simulink model "SimulationModel"  (R2019b)
settings: Solver=FixedStepAuto  StartTime=0.0  StopTime=simStopTime  FixedStep=Ts  RelTol=1e-3
PostLoadFcn:
  | init
values from neighbouring files (symbols this model uses):
  total_vehicles = evalin('base','total_vehicles')    [VehicleLogicSimulator.m]
  x0 = evalin('base','x0')    [VehicleLogicSimulator.m]
  y0 = evalin('base','y0')    [VehicleLogicSimulator.m]
  yaw0 = evalin('base','yaw0')    [VehicleLogicSimulator.m]
undefined symbols (not defined in the file or in its folder): Cf, Cr, index_show_car, Iz, lf, longitudinal_velocity, lr, m, position, tau, Ts, v0, velocity, yaw_angle, yaw_rate
libraries: autolibshared x3, drivingscenarioandsensors x1, simulink_extras x1
settings Model: Creator=The MathWorks, Inc.  LastModifiedBy=curtm
settings DataIOCC: ReturnWorkspaceOutputs=off
settings DebuggingCC: ParameterPrecisionLossMsg=none  PregeneratedLibrarySubsystemCodeDiagnostic=none  ArithmeticOperatorsInVariantConditions=warning
settings HardwareCC: ProdLongLongMode=on
settings SFSimCC: SimUseLocalCustomCode=off  CustomCodeUndefinedFunction=UseInterfaceOnly
settings RTWCC: RTWUseLocalCustomCode=off

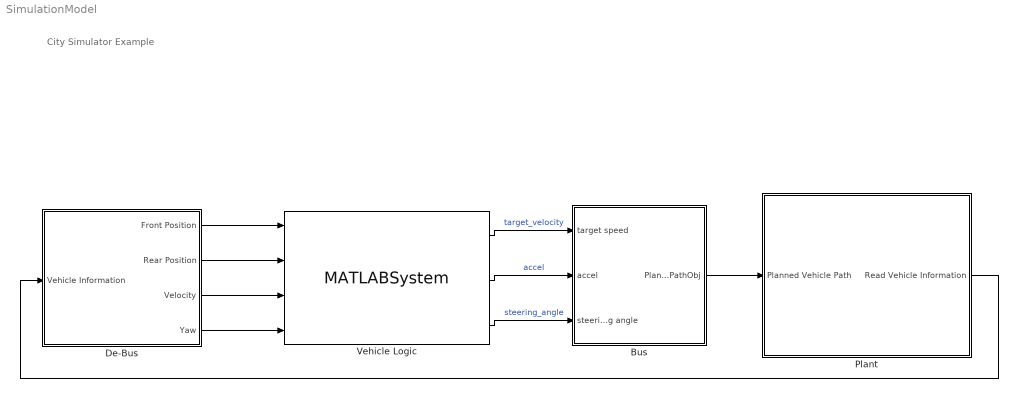
== system SimulationModel ==
  note: City Simulator Example
  Bus : Subsystem
  De-Bus : Subsystem
  Plant : Subsystem
  Vehicle Logic : MATLABSystem  System=VehicleLogicMatlabSystem  SimulateUsing=Code generation
      mask Type: VehicleLogicMatlabSystem
      mask Display:
      | disp('VehicleLogicMatlabSystem');
      | port_label('input',1,'front_pos');
      | port_label('input',2,'rear_pos');
      | port_label('input',3,'velocities');
      | port_label('input',4,'yaws');
      | port_label('output',1,'target_speed');
      | port_label('output',2,'accel');
      | port_label('output',3,'streering_angle');
  wires:
  Bus/1(PlannedVehiclePathObj) -> Plant/1(Planned Vehicle Path)
  Vehicle Logic/1 -> Bus/1(target speed)  "target_velocity"
  Vehicle Logic/2 -> Bus/2(accel)  "accel"
  Vehicle Logic/3 -> Bus/3(steering angle)  "steering_angle"
  De-Bus/2(Rear Position) -> Vehicle Logic/2
  De-Bus/3(Velocity) -> Vehicle Logic/3
  De-Bus/4(Yaw) -> Vehicle Logic/4
  Plant/1(Read Vehicle Information) -> De-Bus/1(Vehicle Information)
  De-Bus/1(Front Position) -> Vehicle Logic/1

== system SimulationModel/Bus ==
  target speed : Inport  OutDataTypeStr=double
  accel : Inport  Port=2  OutDataTypeStr=double
  steering angle : Inport  Port=3  OutDataTypeStr=double
  Planned Vehicle Path From Index 1 : Subsystem  mask{index=1, size=total_vehicles}
      mask prompts: index "Which element of the array?"; size "How many AVs are there?"
  Planned Vehicle Path From Index 2 : Subsystem  mask{index=2, size=total_vehicles}
      mask prompts: index "Which element of the array?"; size "How many AVs are there?"
  Vector Concatenate : Concatenate
  PlannedVehiclePathObj : Outport  OutDataTypeStr=Bus: PlannedVehicleDynamics
  wires:
  Vector Concatenate/1 -> PlannedVehiclePathObj/1
  Planned Vehicle Path From Index 1/1(PlannedVehiclePathObj) -> Vector Concatenate/1
  target speed/1 -> Planned Vehicle Path From Index 2/1(target_speed), Planned Vehicle Path From Index 1/1(target_speed)
  accel/1 -> Planned Vehicle Path From Index 2/2(accel), Planned Vehicle Path From Index 1/2(accel)
  steering angle/1 -> Planned Vehicle Path From Index 2/3(steering_angle), Planned Vehicle Path From Index 1/3(steering_angle)
  Planned Vehicle Path From Index 2/1(PlannedVehiclePathObj) -> Vector Concatenate/2

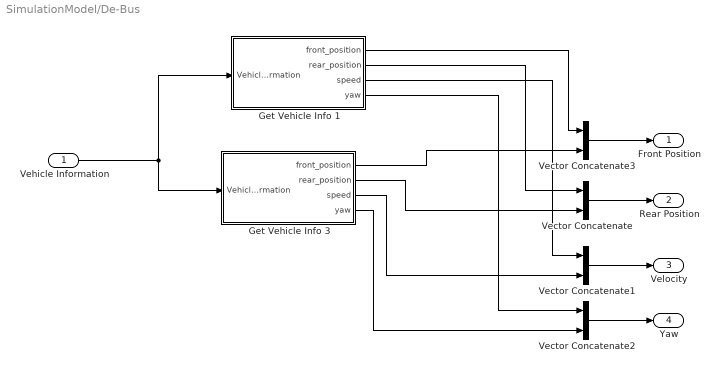
== system SimulationModel/De-Bus ==
  Vehicle Information : Inport
  Get Vehicle Info 1 : Subsystem  mask{index=1, size=total_vehicles}
  Get Vehicle Info 3 : Subsystem  mask{index=2, size=total_vehicles}
  Vector Concatenate{,1..3} (4 alike) : Concatenate
  Front Position : Outport
  Rear Position : Outport  Port=2
  Velocity : Outport  Port=3
  Yaw : Outport  Port=4
  wires:
  Vector Concatenate/1 -> Rear Position/1
  Vector Concatenate1/1 -> Velocity/1
  Vehicle Information/1 -> Get Vehicle Info 3/1(Vehicle Information), Get Vehicle Info 1/1(Vehicle Information)
  Get Vehicle Info 1/2(rear_position) -> Vector Concatenate/1
  Get Vehicle Info 1/3(speed) -> Vector Concatenate1/1
  Get Vehicle Info 3/2(rear_position) -> Vector Concatenate/2
  Get Vehicle Info 3/3(speed) -> Vector Concatenate1/2
  Vector Concatenate2/1 -> Yaw/1
  Get Vehicle Info 1/4(yaw) -> Vector Concatenate2/1
  Get Vehicle Info 3/4(yaw) -> Vector Concatenate2/2
  Get Vehicle Info 1/1(front_position) -> Vector Concatenate3/1
  Vector Concatenate3/1 -> Front Position/1
  Get Vehicle Info 3/1(front_position) -> Vector Concatenate3/2

== system SimulationModel/Plant ==
  note: Vehicle and Environment
  Planned Vehicle Path : Inport  OutDataTypeStr=Bus: PlannedVehicleDynamics  SampleTime=Ts
  Pack for Scenario Reader : Subsystem
  Scenario Reader : drivingscenarioandsensors/Scenario Reader  ScenarioSource=From file  ScenarioFileName=MarcCity.mat  ScenarioVariableName=scenario  OutputCoordinateSystem=Vehicle coordinates  EgoVehicleSource=Input port  EgoVehicleActorID=1  SampleTime=Ts  LaneBoundaryOutput=Ego vehicle lane boundaries  LaneBoundaryDistance=0:0.5:60  LaneBoundaryLocation=Inner edge of lane markings  BusNameSource=Auto  BusName=BusActors  BusName2Source=Auto  BusName2=BusLaneBoundaries  SimulateUsing=Interpreted execution
      settings: SourceProductName=Automated Driving Toolbox
  Terminator : Terminator
  Terminator1 : Terminator
  Vehicle Simulation : Subsystem
  Vehicle Simulation1 : Subsystem  Commented=on  TreatAsAtomicUnit=on
  Read Vehicle Information : Outport  SampleTime=Ts
  wires:
  Planned Vehicle Path/1 -> Vehicle Simulation/1(Planned Vehicle Dynamics)
  Vehicle Simulation/1(Next Vehicle Dynamics) -> Pack for Scenario Reader/1(Bus), Read Vehicle Information/1
  Scenario Reader/1 -> Terminator/1
  Scenario Reader/2 -> Terminator1/1
  Pack for Scenario Reader/1(Scenario Reader Struct) -> Scenario Reader/1

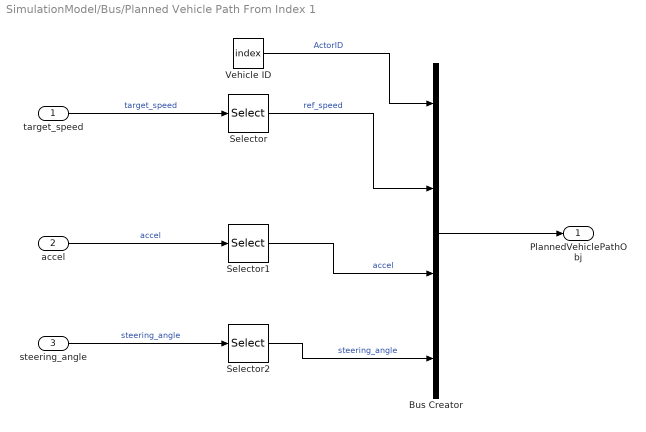
== system SimulationModel/Bus/Planned Vehicle Path From Index 1 ==
  target_speed : Inport
  accel : Inport  Port=2
  steering_angle : Inport  Port=3
  Bus Creator : BusCreator  Inputs=4  OutDataTypeStr=Bus: PlannedVehicleDynamics  NonVirtualBus=on
  Selector : Selector  NumberOfDimensions=2  InputPortWidth=size  IndexOptions=Index vector (dialog),Index vector (dialog)  Indices=index,1  OutputSizes=1,1
  Selector1 : Selector  NumberOfDimensions=2  InputPortWidth=size  IndexOptions=Index vector (dialog),Index vector (dialog)  Indices=index,1  OutputSizes=1,1
  Selector2 : Selector  NumberOfDimensions=2  InputPortWidth=size  IndexOptions=Index vector (dialog),Index vector (dialog)  Indices=index,1  OutputSizes=1,1
  Vehicle ID : Constant  Value=index
  PlannedVehiclePathObj : Outport
  wires:
  target_speed/1 -> Selector/1  "target_speed"
  steering_angle/1 -> Selector2/1  "steering_angle"
  accel/1 -> Selector1/1  "accel"
  Selector/1 -> Bus Creator/2  "ref_speed"
  Selector1/1 -> Bus Creator/3  "accel"
  Selector2/1 -> Bus Creator/4  "steering_angle"
  Bus Creator/1 -> PlannedVehiclePathObj/1
  Vehicle ID/1 -> Bus Creator/1  "ActorID"

== system SimulationModel/Bus/Planned Vehicle Path From Index 2 ==
  target_speed : Inport
  accel : Inport  Port=2
  steering_angle : Inport  Port=3
  Bus Creator : BusCreator  Inputs=4  OutDataTypeStr=Bus: PlannedVehicleDynamics  NonVirtualBus=on
  Selector : Selector  InputPortWidth=size  IndexOptions=Index vector (dialog)  Indices=index  OutputSizes=1
  Selector3 : Selector  InputPortWidth=size  IndexOptions=Index vector (dialog)  Indices=index  OutputSizes=1
  Selector4 : Selector  InputPortWidth=size  IndexOptions=Index vector (dialog)  Indices=index  OutputSizes=1
  Vehicle ID : Constant  Value=index
  PlannedVehiclePathObj : Outport
  wires:
  target_speed/1 -> Selector/1  "target_speed"
  steering_angle/1 -> Selector4/1  "steering_angle"
  accel/1 -> Selector3/1  "accel"
  Selector/1 -> Bus Creator/2  "ref_speed"
  Selector3/1 -> Bus Creator/3  "accel"
  Selector4/1 -> Bus Creator/4  "steering_angle"
  Bus Creator/1 -> PlannedVehiclePathObj/1
  Vehicle ID/1 -> Bus Creator/1  "ActorID"

== system SimulationModel/De-Bus/Get Vehicle Info 1 ==
  Vehicle Information : Inport  OutDataTypeStr=Bus: NextVehicleDynamics
  Bus Selector : BusSelector  OutputSignals=front_position,rear_position,longitudinal_velocity,yaw_angle
  Selector : Selector  InputPortWidth=size  IndexOptions=Index vector (dialog)  Indices=[index]  OutputSizes=1
  front_position : Outport
  rear_position : Outport  Port=2
  speed : Outport  Port=3
  yaw : Outport  Port=4
  wires:
  Vehicle Information/1 -> Selector/1
  Selector/1 -> Bus Selector/1
  Bus Selector/2 -> rear_position/1  "<rear_position>"
  Bus Selector/3 -> speed/1  "<longitudinal_velocity>"
  Bus Selector/4 -> yaw/1  "<yaw_angle>"
  Bus Selector/1 -> front_position/1  "<front_position>"

== system SimulationModel/De-Bus/Get Vehicle Info 3 ==
  Vehicle Information : Inport  OutDataTypeStr=Bus: NextVehicleDynamics
  Bus Selector : BusSelector  OutputSignals=front_position,rear_position,longitudinal_velocity,yaw_angle
  Selector : Selector  InputPortWidth=size  IndexOptions=Index vector (dialog)  Indices=[index]  OutputSizes=1
  front_position : Outport
  rear_position : Outport  Port=2
  speed : Outport  Port=3
  yaw : Outport  Port=4
  wires:
  Vehicle Information/1 -> Selector/1
  Selector/1 -> Bus Selector/1
  Bus Selector/2 -> rear_position/1  "<rear_position>"
  Bus Selector/3 -> speed/1  "<longitudinal_velocity>"
  Bus Selector/4 -> yaw/1  "<yaw_angle>"
  Bus Selector/1 -> front_position/1  "<front_position>"

== system SimulationModel/Plant/Pack for Scenario Reader ==
  Bus : Inport
  Clock : Clock  Commented=on
  MATLAB Function : MATLAB Function  Commented=on  TreatAsAtomicUnit=on
  Multiport Switch : MultiPortSwitch  Inputs=2
  Pack bus : Subsystem  mask{index=1, size=total_vehicles}
  Pack bus1 : Subsystem  mask{index=2, size=total_vehicles}
  Selector : Constant  Value=index_show_car
  Terminator : Terminator  Commented=on
  Scenario Reader Struct : Outport
  wires:
  Bus/1 -> Pack bus1/1(Bus), Pack bus/1(Bus)
  Pack bus/1(Scenario Reader Struct) -> Multiport Switch/2
  Multiport Switch/1 -> Scenario Reader Struct/1
  Pack bus1/1(Scenario Reader Struct) -> Multiport Switch/3
  Selector/1 -> Multiport Switch/1
  Clock/1 -> MATLAB Function/3(simTime)
  MATLAB Function/1(Actors) -> Terminator/1

== system SimulationModel/Plant/Vehicle Simulation ==
  Planned Vehicle Dynamics : Inport
  Vector Concatenate : Concatenate
  Vehicle 1 Simulation : Subsystem  mask{index=1, size=total_vehicles}
  Vehicle 2 Simulation : Subsystem  mask{index=2, size=total_vehicles}
  Next Vehicle Dynamics : Outport
  wires:
  Planned Vehicle Dynamics/1 -> Vehicle 2 Simulation/1(InBus), Vehicle 1 Simulation/1(InBus)
  Vehicle 1 Simulation/1(outBus) -> Vector Concatenate/1
  Vector Concatenate/1 -> Next Vehicle Dynamics/1
  Vehicle 2 Simulation/1(outBus) -> Vector Concatenate/2

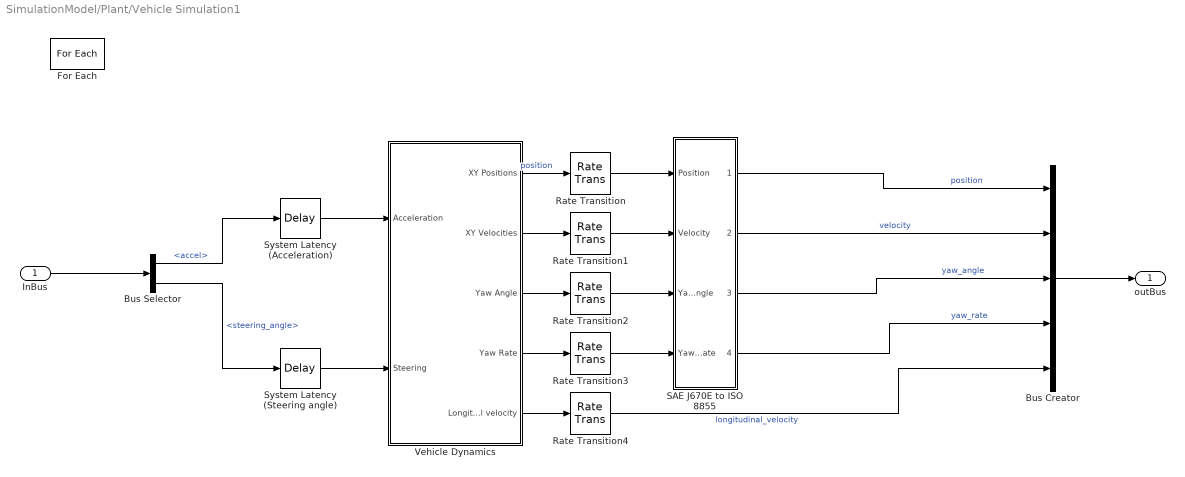
== system SimulationModel/Plant/Vehicle Simulation1 ==
  InBus : Inport  OutDataTypeStr=Bus: PlannedVehicleDynamics  PortDimensions=1  SampleTime=Ts  Partition=on  PartitionDimension=1  PartitionWidth=1  PartitionOffset=0
  Bus Creator : BusCreator  Inputs=position,velocity,yaw_angle,yaw_rate,longitudinal_velocity  OutDataTypeStr=Bus: NextVehicleDynamics  NonVirtualBus=on
  Bus Selector : BusSelector  OutputSignals=accel,steering_angle
  For Each : ForEach  DisableCoverage=on
  Rate Transition{,1..4} (5 alike) : RateTransition  OutPortSampleTime=Ts
  SAE J670E to ISO 8855 : Subsystem
  System Latency (Acceleration) : TransportDelay  DelayTime=Ts
  System Latency (Steering angle) : TransportDelay  DelayTime=Ts
  Vehicle Dynamics : Subsystem  VariantControl=Variant2
  outBus : Outport  OutDataTypeStr=Bus: NextVehicleDynamics  SampleTime=Ts  ConcatenationDimension=1
  wires:
  System Latency (Steering angle)/1 -> Vehicle Dynamics/2(Steering)
  System Latency (Acceleration)/1 -> Vehicle Dynamics/1(Acceleration)
  Vehicle Dynamics/1(XY Positions) -> Rate Transition/1  "position"
  Rate Transition/1 -> SAE J670E to ISO 8855/1(Position)
  Vehicle Dynamics/5(Longitudinal velocity) -> Rate Transition4/1
  SAE J670E to ISO 8855/2(2) -> Bus Creator/2  "velocity"
  Vehicle Dynamics/3(Yaw Angle) -> Rate Transition2/1
  SAE J670E to ISO 8855/1(1) -> Bus Creator/1  "position"
  Rate Transition4/1 -> Bus Creator/5  "longitudinal_velocity"
  SAE J670E to ISO 8855/4(4) -> Bus Creator/4  "yaw_rate"
  Rate Transition3/1 -> SAE J670E to ISO 8855/4(Yaw Rate)
  Rate Transition1/1 -> SAE J670E to ISO 8855/2(Velocity)
  SAE J670E to ISO 8855/3(3) -> Bus Creator/3  "yaw_angle"
  Vehicle Dynamics/2(XY Velocities) -> Rate Transition1/1
  Vehicle Dynamics/4(Yaw Rate) -> Rate Transition3/1
  Rate Transition2/1 -> SAE J670E to ISO 8855/3(Yaw Angle)
  InBus/1 -> Bus Selector/1
  Bus Selector/1 -> System Latency (Acceleration)/1  "<accel>"
  Bus Selector/2 -> System Latency (Steering angle)/1  "<steering_angle>"
  Bus Creator/1 -> outBus/1

== system SimulationModel/Plant/Pack for Scenario Reader/Pack bus ==
  Bus : Inport
  Bus Selector : BusSelector  OutputSignals=rear_position,velocity,yaw_angle,yaw_rate,longitudinal_velocity
  Constant : Constant  Value=index
  Pack Ego Actor : MATLAB Function  TreatAsAtomicUnit=on  SystemSampleTime=Ts
  Selector : Selector  InputPortWidth=size  IndexOptions=Index vector (dialog)  Indices=index  OutputSizes=1
  Terminator : Terminator
  Scenario Reader Struct : Outport
  wires:
  Constant/1 -> Pack Ego Actor/1(actorID)
  Bus Selector/4 -> Pack Ego Actor/5(yawRate)  "<yaw_rate>"
  Bus Selector/3 -> Pack Ego Actor/4(yaw)  "<yaw_angle>"
  Bus Selector/2 -> Pack Ego Actor/3(vel)  "<velocity>"
  Bus Selector/5 -> Terminator/1  "<longitudinal_velocity>"
  Pack Ego Actor/1(a) -> Scenario Reader Struct/1
  Selector/1 -> Bus Selector/1  "bus"
  Bus/1 -> Selector/1
  Bus Selector/1 -> Pack Ego Actor/2(pos)  "<rear_position>"

== system SimulationModel/Plant/Pack for Scenario Reader/Pack bus1 ==
  Bus : Inport
  Bus Selector : BusSelector  OutputSignals=rear_position,velocity,yaw_angle,yaw_rate,longitudinal_velocity
  Constant : Constant  Value=index
  Pack Ego Actor : MATLAB Function  TreatAsAtomicUnit=on  SystemSampleTime=Ts
  Selector : Selector  InputPortWidth=size  IndexOptions=Index vector (dialog)  Indices=index  OutputSizes=1
  Terminator : Terminator
  Scenario Reader Struct : Outport
  wires:
  Constant/1 -> Pack Ego Actor/1(actorID)
  Bus Selector/4 -> Pack Ego Actor/5(yawRate)  "<yaw_rate>"
  Bus Selector/3 -> Pack Ego Actor/4(yaw)  "<yaw_angle>"
  Bus Selector/2 -> Pack Ego Actor/3(vel)  "<velocity>"
  Bus Selector/5 -> Terminator/1  "<longitudinal_velocity>"
  Pack Ego Actor/1(a) -> Scenario Reader Struct/1
  Bus Selector/1 -> Pack Ego Actor/2(pos)  "<rear_position>"
  Selector/1 -> Bus Selector/1  "bus"
  Bus/1 -> Selector/1

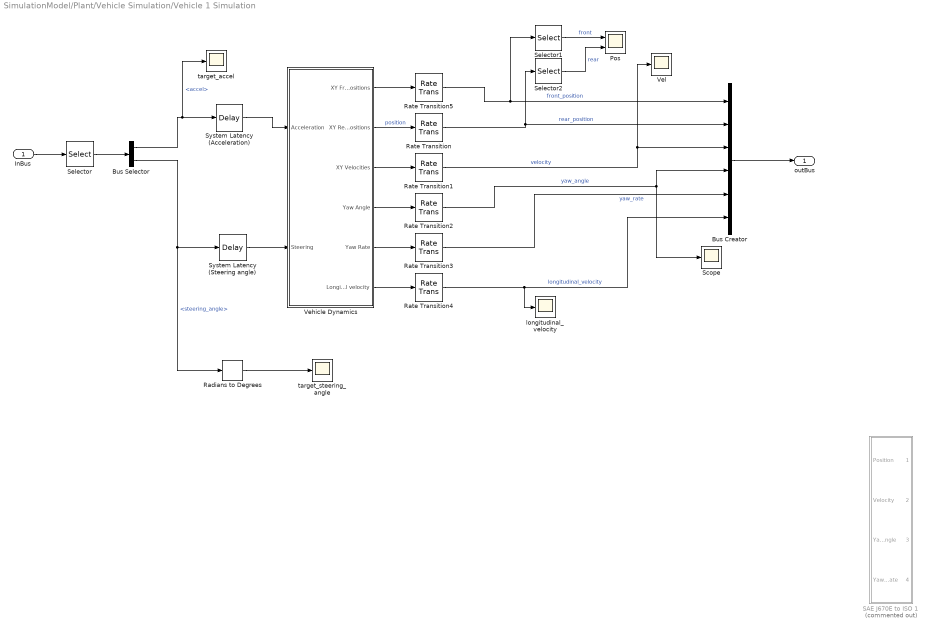
== system SimulationModel/Plant/Vehicle Simulation/Vehicle 1 Simulation ==
  InBus : Inport  OutDataTypeStr=Bus: PlannedVehicleDynamics  PortDimensions=1  SampleTime=Ts
  Bus Creator : BusCreator  Inputs=6  OutDataTypeStr=Bus: NextVehicleDynamics  NonVirtualBus=on
  Bus Selector : BusSelector  OutputSignals=accel,steering_angle
  Pos : Scope  NumInputPorts=2
  Radians to Degrees : simulink_extras/Transformations/Radians to Degrees
  Rate Transition{,1..5} (6 alike) : RateTransition  OutPortSampleTime=Ts
  SAE J670E to ISO 1 : Subsystem  Commented=on
  Scope : Scope
  Selector : Selector  InputPortWidth=size  IndexOptions=Index vector (dialog)  Indices=index  OutputSizes=1
  Selector1 : Selector  InputPortWidth=2  IndexOptions=Index vector (dialog)  Indices=2  OutputSizes=1
  Selector2 : Selector  InputPortWidth=2  IndexOptions=Index vector (dialog)  Indices=2  OutputSizes=1
  System Latency (Acceleration) : TransportDelay  DelayTime=Ts
  System Latency (Steering angle) : TransportDelay  DelayTime=Ts
  Vehicle Dynamics : Subsystem  VariantControl=Variant2
  Vel : Scope
  longitudinal_velocity : Scope
  target_accel : Scope
  target_steering_angle : Scope
  outBus : Outport  OutDataTypeStr=Bus: NextVehicleDynamics  SampleTime=Ts
  wires:
  Rate Transition2/1 -> Scope/1, Bus Creator/4  "yaw_angle"
  Rate Transition4/1 -> Bus Creator/6, longitudinal_velocity/1  "longitudinal_velocity"
  Vehicle Dynamics/6(Longitudinal velocity) -> Rate Transition4/1
  Vehicle Dynamics/4(Yaw Angle) -> Rate Transition2/1
  Vehicle Dynamics/3(XY Velocities) -> Rate Transition1/1
  Vehicle Dynamics/2(XY Rear Positions) -> Rate Transition/1  "position"
  Bus Creator/1 -> outBus/1
  Bus Selector/2 -> Radians to Degrees/1, System Latency (Steering angle)/1  "<steering_angle>"
  Rate Transition/1 -> Selector2/1, Bus Creator/2  "rear_position"
  InBus/1 -> Selector/1
  Rate Transition3/1 -> Bus Creator/5  "yaw_rate"
  System Latency (Steering angle)/1 -> Vehicle Dynamics/2(Steering)
  System Latency (Acceleration)/1 -> Vehicle Dynamics/1(Acceleration)
  Rate Transition1/1 -> Vel/1, Bus Creator/3  "velocity"
  Vehicle Dynamics/5(Yaw Rate) -> Rate Transition3/1
  Bus Selector/1 -> target_accel/1, System Latency (Acceleration)/1  "<accel>"
  Selector/1 -> Bus Selector/1
  Vehicle Dynamics/1(XY Front Positions) -> Rate Transition5/1
  Rate Transition5/1 -> Selector1/1, Bus Creator/1  "front_position"
  Radians to Degrees/1 -> target_steering_angle/1
  Selector1/1 -> Pos/1  "front"
  Selector2/1 -> Pos/2  "rear"

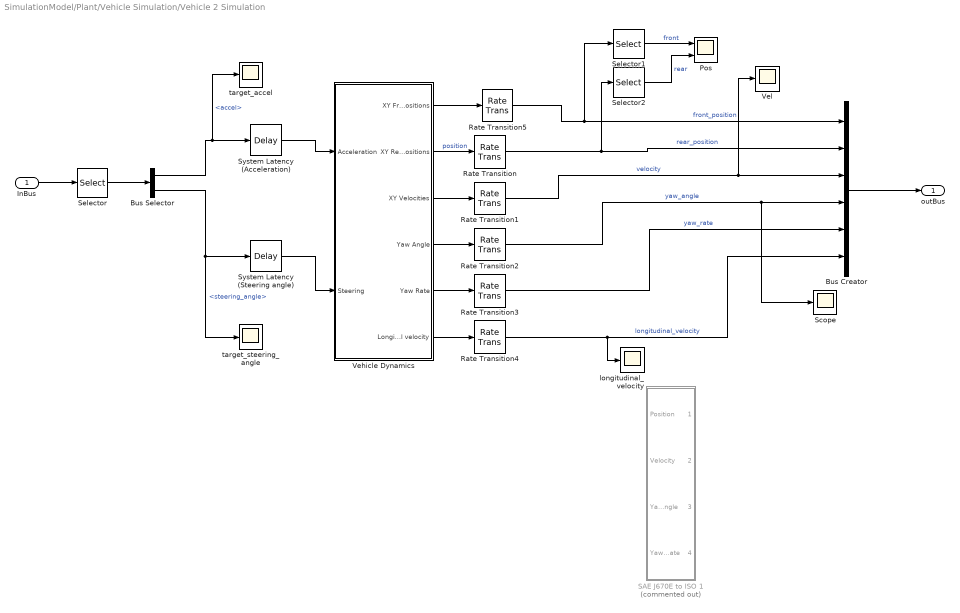
== system SimulationModel/Plant/Vehicle Simulation/Vehicle 2 Simulation ==
  InBus : Inport  OutDataTypeStr=Bus: PlannedVehicleDynamics  PortDimensions=1  SampleTime=Ts
  Bus Creator : BusCreator  Inputs=6  OutDataTypeStr=Bus: NextVehicleDynamics  NonVirtualBus=on
  Bus Selector : BusSelector  OutputSignals=accel,steering_angle
  Pos : Scope  NumInputPorts=2
  Rate Transition{,1..5} (6 alike) : RateTransition  OutPortSampleTime=Ts
  SAE J670E to ISO 1 : Subsystem  Commented=on
  Scope : Scope
  Selector : Selector  InputPortWidth=size  IndexOptions=Index vector (dialog)  Indices=index  OutputSizes=1
  Selector1 : Selector  InputPortWidth=2  IndexOptions=Index vector (dialog)  Indices=2  OutputSizes=1
  Selector2 : Selector  InputPortWidth=2  IndexOptions=Index vector (dialog)  Indices=2  OutputSizes=1
  System Latency (Acceleration) : TransportDelay  DelayTime=Ts
  System Latency (Steering angle) : TransportDelay  DelayTime=Ts
  Vehicle Dynamics : Subsystem  VariantControl=Variant2
  Vel : Scope
  longitudinal_velocity : Scope
  target_accel : Scope
  target_steering_angle : Scope
  outBus : Outport  OutDataTypeStr=Bus: NextVehicleDynamics  SampleTime=Ts
  wires:
  Rate Transition2/1 -> Scope/1, Bus Creator/4  "yaw_angle"
  Rate Transition4/1 -> Bus Creator/6, longitudinal_velocity/1  "longitudinal_velocity"
  Vehicle Dynamics/6(Longitudinal velocity) -> Rate Transition4/1
  Vehicle Dynamics/4(Yaw Angle) -> Rate Transition2/1
  Vehicle Dynamics/3(XY Velocities) -> Rate Transition1/1
  Vehicle Dynamics/2(XY Rear Positions) -> Rate Transition/1  "position"
  Bus Creator/1 -> outBus/1
  Bus Selector/2 -> target_steering_angle/1, System Latency (Steering angle)/1  "<steering_angle>"
  InBus/1 -> Selector/1
  Rate Transition3/1 -> Bus Creator/5  "yaw_rate"
  System Latency (Steering angle)/1 -> Vehicle Dynamics/2(Steering)
  System Latency (Acceleration)/1 -> Vehicle Dynamics/1(Acceleration)
  Rate Transition1/1 -> Vel/1, Bus Creator/3  "velocity"
  Vehicle Dynamics/5(Yaw Rate) -> Rate Transition3/1
  Bus Selector/1 -> target_accel/1, System Latency (Acceleration)/1  "<accel>"
  Selector/1 -> Bus Selector/1
  Vehicle Dynamics/1(XY Front Positions) -> Rate Transition5/1
  Rate Transition5/1 -> Selector1/1, Bus Creator/1  "front_position"
  Selector1/1 -> Pos/1  "front"
  Rate Transition/1 -> Selector2/1, Bus Creator/2  "rear_position"
  Selector2/1 -> Pos/2  "rear"

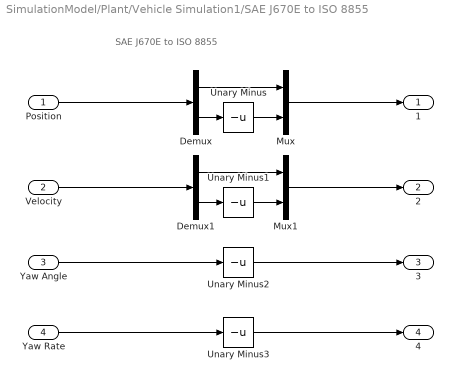
== system SimulationModel/Plant/Vehicle Simulation1/SAE J670E to ISO 8855 ==
  note: SAE J670E to ISO 8855
  Position : Inport  OutDataTypeStr=double  Unit=m
  Velocity : Inport  Port=2  OutDataTypeStr=double  Unit=m/s
  Yaw Angle : Inport  Port=3  OutDataTypeStr=double  Unit=deg
  Yaw Rate : Inport  Port=4  OutDataTypeStr=double  Unit=deg/s
  Demux : Demux  Outputs=2
  Demux1 : Demux  Outputs=2
  Mux : Mux  Inputs=2
  Mux1 : Mux  Inputs=2
  Unary Minus{,1..3} (4 alike) : UnaryMinus
  1 : Outport  OutDataTypeStr=double  VectorParamsAs1DForOutWhenUnconnected=off
  2 : Outport  Port=2  OutDataTypeStr=double  VectorParamsAs1DForOutWhenUnconnected=off
  3 : Outport  Port=3  OutDataTypeStr=double  PortDimensions=1  VectorParamsAs1DForOutWhenUnconnected=off
  4 : Outport  Port=4  OutDataTypeStr=double  PortDimensions=1  VectorParamsAs1DForOutWhenUnconnected=off
  wires:
  Yaw Rate/1 -> Unary Minus3/1
  Yaw Angle/1 -> Unary Minus2/1
  Demux/1 -> Mux/1
  Demux/2 -> Unary Minus/1
  Unary Minus/1 -> Mux/2
  Unary Minus1/1 -> Mux1/2
  Demux1/2 -> Unary Minus1/1
  Demux1/1 -> Mux1/1
  Mux1/1 -> 2/1
  Mux/1 -> 1/1
  Position/1 -> Demux/1
  Velocity/1 -> Demux1/1
  Unary Minus2/1 -> 3/1
  Unary Minus3/1 -> 4/1

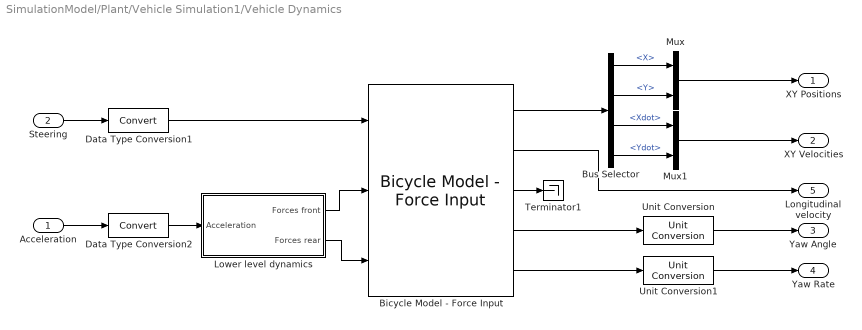
== system SimulationModel/Plant/Vehicle Simulation1/Vehicle Dynamics ==
  Acceleration : Inport  Unit=m/s^2
  Steering : Inport  Port=2  Unit=rad
  Bicycle Model - Force Input : autolibshared/Bicycle Model - Force Input  trackMode=Single (bicycle)  inputMode=External longitudinal forces  frontSteerMode=on  rearSteerMode=off  windMode=off  muMode=off  extFMode=off  extMMode=off  aMode=3  NF=2  NR=2  m=m  a=lf  b=lr  h=0.35  X_o=x0_ego  xdot_o=v0_ego  CalphaMode=off  sigmaMode=on  w=[1.4,1.4]  Cy_f=Cf  Cy_r=Cr  sigma_f=.1  sigma_r=.1  alpha_f_brk=[-.1 .1]  Cy_f_data=[-9e3 9e3]  alpha_r_brk=[-.1 .1]  Cy_r_data=[-9e3 9e3]  Y_o=y0_ego  ydot_o=0  Izz=Iz  psi_o=yaw0_ego  r_o=0  Af=0  Cd=.3  Cl=.1  Cpm=.1  beta_w=[0:0.01:0.3]  Cs=[0:0.03:0.9]  Cym=[0:0.01:0.3]  Pabs=101325  Tair=273  g=9.81  mu=1  xdot_tol=.01  Fznom=5000  Fxtire_sat=1e6  Fytire_sat=1e6  longOff=0  latOff=0  vertOff=0
      settings: SourceProductName=Powertrain Blockset  SourceProductBaseCode=PW
  Bus Selector : BusSelector  OutputSignals=InertFrm.FrntAxl.Disp.X,InertFrm.FrntAxl.Disp.Y,InertFrm.FrntAxl.Vel.Xdot,InertFrm.FrntAxl.Vel.Ydot
  Data Type Conversion1 : DataTypeConversion
  Data Type Conversion2 : DataTypeConversion
  Lower level dynamics : Subsystem
  Mux : Mux  Inputs=2
  Mux1 : Mux  Inputs=2
  Terminator1 : Terminator
  Unit Conversion : UnitConversion  OutputType=Inherit: Inherit via back propagation
  Unit Conversion1 : UnitConversion  OutputType=Inherit: Inherit via back propagation
  XY Positions : Outport  Unit=m  VectorParamsAs1DForOutWhenUnconnected=off
  XY Velocities : Outport  Port=2  Unit=m/s  VectorParamsAs1DForOutWhenUnconnected=off
  Yaw Angle : Outport  Port=3  Unit=deg  VectorParamsAs1DForOutWhenUnconnected=off
  Yaw Rate : Outport  Port=4  Unit=degree/s  VectorParamsAs1DForOutWhenUnconnected=off
  Longitudinal velocity : Outport  Port=5  VectorParamsAs1DForOutWhenUnconnected=off
  wires:
  Lower level dynamics/2(Forces rear) -> Bicycle Model - Force Input/3
  Lower level dynamics/1(Forces front) -> Bicycle Model - Force Input/2
  Data Type Conversion2/1 -> Lower level dynamics/1(Acceleration)
  Data Type Conversion1/1 -> Bicycle Model - Force Input/1
  Acceleration/1 -> Data Type Conversion2/1
  Steering/1 -> Data Type Conversion1/1
  Bus Selector/1 -> Mux/1  "<X>"
  Unit Conversion/1 -> Yaw Angle/1
  Bicycle Model - Force Input/5 -> Unit Conversion1/1
  Bus Selector/4 -> Mux1/2  "<Ydot>"
  Bicycle Model - Force Input/4 -> Unit Conversion/1
  Bus Selector/2 -> Mux/2  "<Y>"
  Bicycle Model - Force Input/2 -> Longitudinal velocity/1
  Bus Selector/3 -> Mux1/1  "<Xdot>"
  Bicycle Model - Force Input/1 -> Bus Selector/1
  Bicycle Model - Force Input/3 -> Terminator1/1
  Mux/1 -> XY Positions/1
  Mux1/1 -> XY Velocities/1
  Unit Conversion1/1 -> Yaw Rate/1

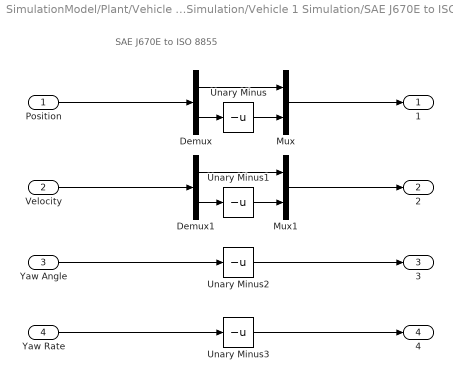
== system SimulationModel/Plant/Vehicle Simulation/Vehicle 1 Simulation/SAE J670E to ISO 1 ==
  note: SAE J670E to ISO 8855
  Position : Inport  OutDataTypeStr=double  Unit=m
  Velocity : Inport  Port=2  OutDataTypeStr=double  Unit=m/s
  Yaw Angle : Inport  Port=3  OutDataTypeStr=double  Unit=deg
  Yaw Rate : Inport  Port=4  OutDataTypeStr=double  Unit=deg/s
  Demux : Demux  Outputs=2
  Demux1 : Demux  Outputs=2
  Mux : Mux  Inputs=2
  Mux1 : Mux  Inputs=2
  Unary Minus{,1..3} (4 alike) : UnaryMinus
  1 : Outport  OutDataTypeStr=double  VectorParamsAs1DForOutWhenUnconnected=off
  2 : Outport  Port=2  OutDataTypeStr=double  VectorParamsAs1DForOutWhenUnconnected=off
  3 : Outport  Port=3  OutDataTypeStr=double  PortDimensions=1  VectorParamsAs1DForOutWhenUnconnected=off
  4 : Outport  Port=4  OutDataTypeStr=double  PortDimensions=1  VectorParamsAs1DForOutWhenUnconnected=off
  wires:
  Yaw Rate/1 -> Unary Minus3/1
  Demux/1 -> Mux/1
  Demux/2 -> Unary Minus/1
  Unary Minus/1 -> Mux/2
  Unary Minus1/1 -> Mux1/2
  Demux1/2 -> Unary Minus1/1
  Demux1/1 -> Mux1/1
  Mux1/1 -> 2/1
  Mux/1 -> 1/1
  Position/1 -> Demux/1
  Velocity/1 -> Demux1/1
  Yaw Angle/1 -> Unary Minus2/1
  Unary Minus3/1 -> 4/1
  Unary Minus2/1 -> 3/1

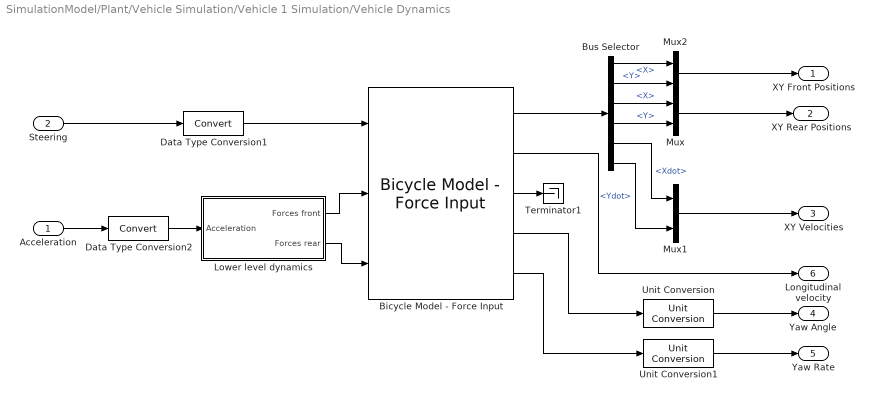
== system SimulationModel/Plant/Vehicle Simulation/Vehicle 1 Simulation/Vehicle Dynamics ==
  Acceleration : Inport  Unit=m/s^2
  Steering : Inport  Port=2  Unit=rad
  Bicycle Model - Force Input : autolibshared/Bicycle Model - Force Input  trackMode=Single (bicycle)  inputMode=External longitudinal forces  frontSteerMode=on  rearSteerMode=off  windMode=off  muMode=off  extFMode=off  extMMode=off  aMode=3  NF=2  NR=2  m=m(index)  a=lf(index)  b=lr(index)  h=0.35  X_o=x0(index)  xdot_o=v0(index)  CalphaMode=off  sigmaMode=on  w=[1.4,1.4]  Cy_f=Cf(index)  Cy_r=Cr(index)  sigma_f=.1  sigma_r=.1  alpha_f_brk=[-.1 .1]  Cy_f_data=[-9e3 9e3]  alpha_r_brk=[-.1 .1]  Cy_r_data=[-9e3 9e3]  Y_o=y0(index)  ydot_o=0  Izz=Iz(index)  psi_o=yaw0(index)  r_o=0  Af=0  Cd=.3  Cl=.1  Cpm=.1  beta_w=[0:0.01:0.3]  Cs=[0:0.03:0.9]  Cym=[0:0.01:0.3]  Pabs=101325  Tair=273  g=9.81  mu=1  xdot_tol=.01  Fznom=5000  Fxtire_sat=1e6  Fytire_sat=1e6  longOff=0  latOff=0  vertOff=0
      settings: SourceProductName=Powertrain Blockset  SourceProductBaseCode=PW
  Bus Selector : BusSelector  OutputSignals=InertFrm.FrntAxl.Disp.X,InertFrm.FrntAxl.Disp.Y,InertFrm.RearAxl.Disp.X,InertFrm.RearAxl.Disp.Y,InertFrm.FrntAxl.Vel.Xdot,InertFrm.FrntAxl.Vel.Ydot
  Data Type Conversion1 : DataTypeConversion
  Data Type Conversion2 : DataTypeConversion
  Lower level dynamics : Subsystem
  Mux : Mux  Inputs=2
  Mux1 : Mux  Inputs=2
  Mux2 : Mux  Inputs=2
  Terminator1 : Terminator
  Unit Conversion : UnitConversion  OutputType=Inherit: Inherit via back propagation
  Unit Conversion1 : UnitConversion  OutputType=Inherit: Inherit via back propagation
  XY Front Positions : Outport  Unit=m  VectorParamsAs1DForOutWhenUnconnected=off
  XY Rear Positions : Outport  Port=2  Unit=m  VectorParamsAs1DForOutWhenUnconnected=off
  XY Velocities : Outport  Port=3  Unit=m/s  VectorParamsAs1DForOutWhenUnconnected=off
  Yaw Angle : Outport  Port=4  Unit=deg  VectorParamsAs1DForOutWhenUnconnected=off
  Yaw Rate : Outport  Port=5  Unit=degree/s  VectorParamsAs1DForOutWhenUnconnected=off
  Longitudinal velocity : Outport  Port=6  VectorParamsAs1DForOutWhenUnconnected=off
  wires:
  Lower level dynamics/2(Forces rear) -> Bicycle Model - Force Input/3
  Lower level dynamics/1(Forces front) -> Bicycle Model - Force Input/2
  Data Type Conversion2/1 -> Lower level dynamics/1(Acceleration)
  Steering/1 -> Data Type Conversion1/1
  Acceleration/1 -> Data Type Conversion2/1
  Unit Conversion/1 -> Yaw Angle/1
  Bicycle Model - Force Input/5 -> Unit Conversion1/1
  Bus Selector/6 -> Mux1/2  "<Ydot>"
  Bicycle Model - Force Input/4 -> Unit Conversion/1
  Bicycle Model - Force Input/2 -> Longitudinal velocity/1
  Bus Selector/5 -> Mux1/1  "<Xdot>"
  Bicycle Model - Force Input/1 -> Bus Selector/1
  Bicycle Model - Force Input/3 -> Terminator1/1
  Mux/1 -> XY Rear Positions/1
  Mux1/1 -> XY Velocities/1
  Unit Conversion1/1 -> Yaw Rate/1
  Data Type Conversion1/1 -> Bicycle Model - Force Input/1
  Mux2/1 -> XY Front Positions/1
  Bus Selector/3 -> Mux/1  "<X>"
  Bus Selector/4 -> Mux/2  "<Y>"
  Bus Selector/1 -> Mux2/1  "<X>"
  Bus Selector/2 -> Mux2/2  "<Y>"

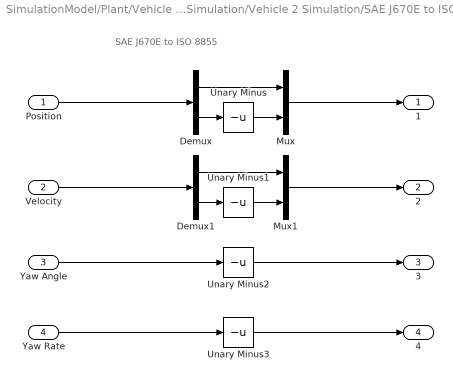
== system SimulationModel/Plant/Vehicle Simulation/Vehicle 2 Simulation/SAE J670E to ISO 1 ==
  note: SAE J670E to ISO 8855
  Position : Inport  OutDataTypeStr=double  Unit=m
  Velocity : Inport  Port=2  OutDataTypeStr=double  Unit=m/s
  Yaw Angle : Inport  Port=3  OutDataTypeStr=double  Unit=deg
  Yaw Rate : Inport  Port=4  OutDataTypeStr=double  Unit=deg/s
  Demux : Demux  Outputs=2
  Demux1 : Demux  Outputs=2
  Mux : Mux  Inputs=2
  Mux1 : Mux  Inputs=2
  Unary Minus{,1..3} (4 alike) : UnaryMinus
  1 : Outport  OutDataTypeStr=double  VectorParamsAs1DForOutWhenUnconnected=off
  2 : Outport  Port=2  OutDataTypeStr=double  VectorParamsAs1DForOutWhenUnconnected=off
  3 : Outport  Port=3  OutDataTypeStr=double  PortDimensions=1  VectorParamsAs1DForOutWhenUnconnected=off
  4 : Outport  Port=4  OutDataTypeStr=double  PortDimensions=1  VectorParamsAs1DForOutWhenUnconnected=off
  wires:
  Yaw Rate/1 -> Unary Minus3/1
  Demux/1 -> Mux/1
  Demux/2 -> Unary Minus/1
  Unary Minus/1 -> Mux/2
  Unary Minus1/1 -> Mux1/2
  Demux1/2 -> Unary Minus1/1
  Demux1/1 -> Mux1/1
  Mux1/1 -> 2/1
  Mux/1 -> 1/1
  Position/1 -> Demux/1
  Velocity/1 -> Demux1/1
  Yaw Angle/1 -> Unary Minus2/1
  Unary Minus3/1 -> 4/1
  Unary Minus2/1 -> 3/1

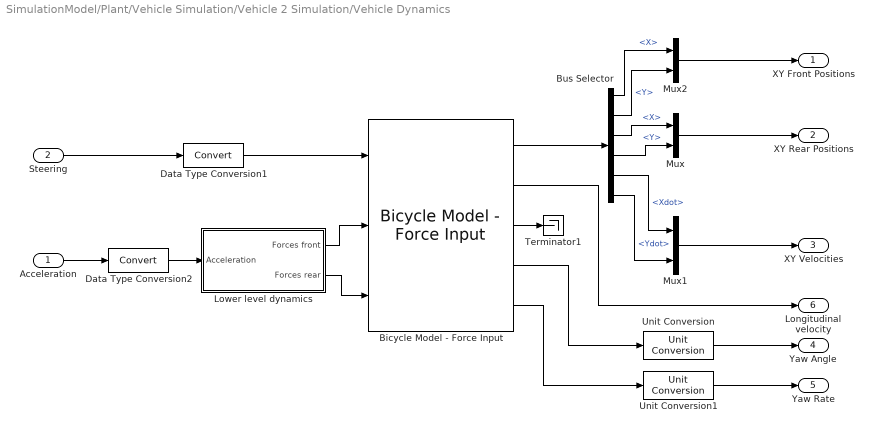
== system SimulationModel/Plant/Vehicle Simulation/Vehicle 2 Simulation/Vehicle Dynamics ==
  Acceleration : Inport  Unit=m/s^2
  Steering : Inport  Port=2  Unit=rad
  Bicycle Model - Force Input : autolibshared/Bicycle Model - Force Input  trackMode=Single (bicycle)  inputMode=External longitudinal forces  frontSteerMode=on  rearSteerMode=off  windMode=off  muMode=off  extFMode=off  extMMode=off  aMode=3  NF=2  NR=2  m=m(index)  a=lf(index)  b=lr(index)  h=0.35  X_o=x0(index)  xdot_o=v0(index)  CalphaMode=off  sigmaMode=on  w=[1.4,1.4]  Cy_f=Cf(index)  Cy_r=Cr(index)  sigma_f=.1  sigma_r=.1  alpha_f_brk=[-.1 .1]  Cy_f_data=[-9e3 9e3]  alpha_r_brk=[-.1 .1]  Cy_r_data=[-9e3 9e3]  Y_o=y0(index)  ydot_o=0  Izz=Iz(index)  psi_o=yaw0(index)  r_o=0  Af=0  Cd=.3  Cl=.1  Cpm=.1  beta_w=[0:0.01:0.3]  Cs=[0:0.03:0.9]  Cym=[0:0.01:0.3]  Pabs=101325  Tair=273  g=9.81  mu=1  xdot_tol=.01  Fznom=5000  Fxtire_sat=1e6  Fytire_sat=1e6  longOff=0  latOff=0  vertOff=0
      settings: SourceProductName=Powertrain Blockset  SourceProductBaseCode=PW
  Bus Selector : BusSelector  OutputSignals=InertFrm.FrntAxl.Disp.X,InertFrm.FrntAxl.Disp.Y,InertFrm.RearAxl.Disp.X,InertFrm.RearAxl.Disp.Y,InertFrm.FrntAxl.Vel.Xdot,InertFrm.FrntAxl.Vel.Ydot
  Data Type Conversion1 : DataTypeConversion
  Data Type Conversion2 : DataTypeConversion
  Lower level dynamics : Subsystem
  Mux : Mux  Inputs=2
  Mux1 : Mux  Inputs=2
  Mux2 : Mux  Inputs=2
  Terminator1 : Terminator
  Unit Conversion : UnitConversion  OutputType=Inherit: Inherit via back propagation
  Unit Conversion1 : UnitConversion  OutputType=Inherit: Inherit via back propagation
  XY Front Positions : Outport  Unit=m  VectorParamsAs1DForOutWhenUnconnected=off
  XY Rear Positions : Outport  Port=2  Unit=m  VectorParamsAs1DForOutWhenUnconnected=off
  XY Velocities : Outport  Port=3  Unit=m/s  VectorParamsAs1DForOutWhenUnconnected=off
  Yaw Angle : Outport  Port=4  Unit=deg  VectorParamsAs1DForOutWhenUnconnected=off
  Yaw Rate : Outport  Port=5  Unit=degree/s  VectorParamsAs1DForOutWhenUnconnected=off
  Longitudinal velocity : Outport  Port=6  VectorParamsAs1DForOutWhenUnconnected=off
  wires:
  Lower level dynamics/2(Forces rear) -> Bicycle Model - Force Input/3
  Lower level dynamics/1(Forces front) -> Bicycle Model - Force Input/2
  Data Type Conversion2/1 -> Lower level dynamics/1(Acceleration)
  Steering/1 -> Data Type Conversion1/1
  Acceleration/1 -> Data Type Conversion2/1
  Bus Selector/1 -> Mux2/1  "<X>"
  Unit Conversion/1 -> Yaw Angle/1
  Bicycle Model - Force Input/5 -> Unit Conversion1/1
  Bus Selector/6 -> Mux1/2  "<Ydot>"
  Bicycle Model - Force Input/4 -> Unit Conversion/1
  Bus Selector/2 -> Mux2/2  "<Y>"
  Bicycle Model - Force Input/2 -> Longitudinal velocity/1
  Bus Selector/5 -> Mux1/1  "<Xdot>"
  Bicycle Model - Force Input/1 -> Bus Selector/1
  Bicycle Model - Force Input/3 -> Terminator1/1
  Mux/1 -> XY Rear Positions/1
  Mux1/1 -> XY Velocities/1
  Unit Conversion1/1 -> Yaw Rate/1
  Data Type Conversion1/1 -> Bicycle Model - Force Input/1
  Bus Selector/3 -> Mux/1  "<X>"
  Bus Selector/4 -> Mux/2  "<Y>"
  Mux2/1 -> XY Front Positions/1

== system SimulationModel/Plant/Vehicle Simulation1/Vehicle Dynamics/Lower level dynamics ==
  Acceleration : Inport
  Gain : Gain  Gain=m
  Gain1 : Gain  Gain=0.5
  Lower level dynamics : TransferFcn  Denominator=[tau 1]
  Forces front : Outport  VectorParamsAs1DForOutWhenUnconnected=off
  Forces rear : Outport  Port=2  VectorParamsAs1DForOutWhenUnconnected=off
  wires:
  Gain/1 -> Gain1/1
  Gain1/1 -> Forces front/1, Forces rear/1
  Acceleration/1 -> Lower level dynamics/1
  Lower level dynamics/1 -> Gain/1

== system SimulationModel/Plant/Vehicle Simulation/Vehicle 1 Simulation/Vehicle Dynamics/Lower level dynamics ==
  Acceleration : Inport
  Gain : Gain  Gain=m
  Gain1 : Gain  Gain=0.5
  Lower level dynamics : TransferFcn  Denominator=[tau 1]
  Forces front : Outport  VectorParamsAs1DForOutWhenUnconnected=off
  Forces rear : Outport  Port=2  VectorParamsAs1DForOutWhenUnconnected=off
  wires:
  Gain/1 -> Gain1/1
  Gain1/1 -> Forces front/1, Forces rear/1
  Acceleration/1 -> Lower level dynamics/1
  Lower level dynamics/1 -> Gain/1

== system SimulationModel/Plant/Vehicle Simulation/Vehicle 2 Simulation/Vehicle Dynamics/Lower level dynamics ==
  Acceleration : Inport
  Gain : Gain  Gain=m
  Gain1 : Gain  Gain=0.5
  Lower level dynamics : TransferFcn  Denominator=[tau 1]
  Forces front : Outport  VectorParamsAs1DForOutWhenUnconnected=off
  Forces rear : Outport  Port=2  VectorParamsAs1DForOutWhenUnconnected=off
  wires:
  Gain/1 -> Gain1/1
  Gain1/1 -> Forces front/1, Forces rear/1
  Acceleration/1 -> Lower level dynamics/1
  Lower level dynamics/1 -> Gain/1

== matlab function SimulationModel/Plant/Pack for Scenario Reader/Pack bus1/Pack Ego Actor ==
  data: actorID input; pos input; a output Bus: BusActors1Actors size=1; vel input; yaw input; yawRate input
function a = packEgo(actorID, pos,vel,yaw,yawRate)
% Pack ego information into a single ego actor bus
%
% Imoprtant note:
% Output is a bus of type BusActorsActors. This is the same bus used by the
% Scenario Reader to output an individual actor. If you change the
% output bus name of Scenario Reader change the output bus name here
% as well by clicking on 'Edit Data' in the menu above.
%ActorIDs = [1, 2];
a = struct();
%coder.varsize('a',[1, 2 * length(BusActors1Actors)]);
a = initStructElement(actorID, pos,vel,yaw,yawRate);
%a(1) = initStructElement(ActorIDs(1), pos,vel,yaw,yawRate);
%a(2) = initStructElement(ActorIDs(2), pos,vel,yaw,yawRate);
end

function s = initStructElement(i,  pos,vel,yaw,yawRate)
    s = struct(...
        'ActorID', i,...
        'Position', [pos(1, 1) pos(2, 1) 0], ...
        'Velocity', [vel(1, 1) vel(2, 1) 0], ...
        'Roll', 0, ...
        'Pitch', 0, ...
        'Yaw', yaw, ...
        'AngularVelocity', [0 0 yawRate]);
end

== matlab function SimulationModel/Plant/Pack for Scenario Reader/Pack bus/Pack Ego Actor ==
  data: actorID input; pos input; a output Bus: BusActors1Actors size=1; vel input; yaw input; yawRate input
function a = packEgo(actorID, pos,vel,yaw,yawRate)
% Pack ego information into a single ego actor bus
%
% Imoprtant note:
% Output is a bus of type BusActorsActors. This is the same bus used by the
% Scenario Reader to output an individual actor. If you change the
% output bus name of Scenario Reader change the output bus name here
% as well by clicking on 'Edit Data' in the menu above.
%ActorIDs = [1, 2];
a = struct();
%coder.varsize('a',[1, 2 * length(BusActors1Actors)]);

a = initStructElement(actorID, pos,vel,yaw,yawRate);
%a(1) = initStructElement(ActorIDs(1), pos,vel,yaw,yawRate);
%a(2) = initStructElement(ActorIDs(2), pos,vel,yaw,yawRate);
end

function s = initStructElement(i,  pos,vel,yaw,yawRate)
    s = struct(...
        'ActorID', i,...
        'Position', [pos(1, 1) pos(2, 1) 0], ...
        'Velocity', [vel(1, 1) vel(2, 1) 0], ...
        'Roll', 0, ...
        'Pitch', 0, ...
        'Yaw', yaw, ...
        'AngularVelocity', [0 0 yawRate]);
end

== matlab function SimulationModel/Plant/Pack for Scenario Reader/MATLAB Function ==
  data: egoActor input; Actors output Bus: BusActors1; cycleActor input; simTime input
function Actors = fcn(egoActor, cycleActor, simTime)
Actors = struct();    
actors = [egoActor, cycleActor];
    actorPoses = driving.scenario.targetsToEgo(actors, egoActor);
    Actors = struct('NumActors', 1, ...
        'Time', simTime, ...
        'Actors', actorPoses');
